simulink subsystem "BLDC_qd_coords"  (R2024a)
settings: Solver=VariableStepAuto  StartTime=0.0  StopTime=10.0  RelTol=1e-3
values from neighbouring files (symbols this model uses):
  Dm = 1e-4    (= 0.0001)    [BLDC_Parameters.m]
  Jt = 1e-3    (= 0.001)    [BLDC_Parameters.m]
  lambda_m = torque_const/(3*P/4)    (= 0.00985)    [BLDC_Parameters.m]
  Lss = Lls + 1.5*Lms    (= 0.0006125)    [BLDC_Parameters.m]
  P = 8    [BLDC_Parameters.m]
  rs = 0.69/2    (= 0.345)    [BLDC_Parameters.m]
  tau_s = 1.06e-3    (= 0.00106)    [BLDC_Parameters.m]
settings Model: Creator=matthewhasman  LastModifiedBy=matthewhasman

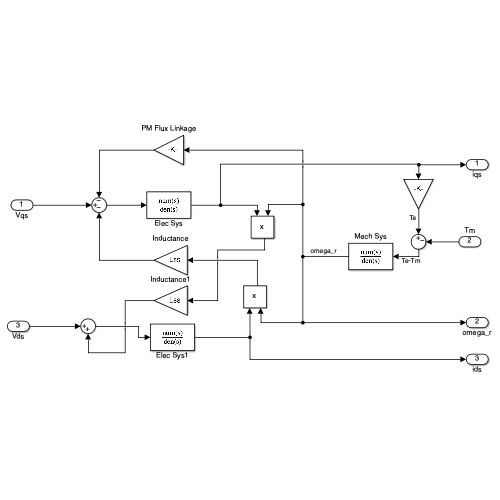
[thumbnail: Simulink's stored preview of the top-level diagram]
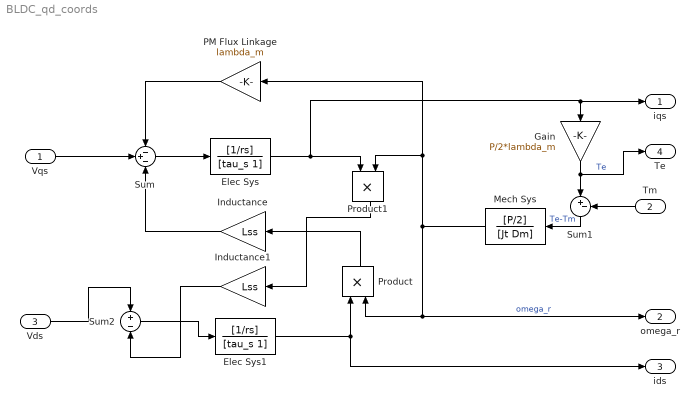
== system BLDC_qd_coords ==
  Vqs : Inport
  Tm : Inport  Port=2
  Vds : Inport  Port=3
  Elec Sys : TransferFcn  Numerator=[1/rs]  Denominator=[tau_s 1]
  Elec Sys1 : TransferFcn  Numerator=[1/rs]  Denominator=[tau_s 1]
  Gain : Gain  Gain=P/2*lambda_m
  Inductance : Gain  Gain=Lss
  Inductance1 : Gain  Gain=Lss
  Mech Sys : TransferFcn  Numerator=[P/2]  Denominator=[Jt Dm]
  PM Flux Linkage : Gain  Gain=lambda_m
  Product : Product
  Product1 : Product
  Sum : Sum  Inputs=-+-
  Sum1 : Sum  Inputs=|+-
  Sum2 : Sum  Inputs=+-
  iqs : Outport
  omega_r : Outport  Port=2
  ids : Outport  Port=3
  Te : Outport  Port=4
  wires:
  Sum/1 -> Elec Sys/1
  Vqs/1 -> Sum/2
  PM Flux Linkage/1 -> Sum/1
  Mech Sys/1 -> Product1/2, PM Flux Linkage/1, omega_r/1, Product/2  "omega_r"
  Inductance/1 -> Sum/3
  Product/1 -> Inductance/1
  Elec Sys/1 -> Product1/1, iqs/1, Gain/1
  Gain/1 -> Sum1/1, Te/1  "Te"
  Tm/1 -> Sum1/2
  Sum1/1 -> Mech Sys/1  "Te-Tm"
  Vds/1 -> Sum2/1
  Product1/1 -> Inductance1/1
  Inductance1/1 -> Sum2/2
  Sum2/1 -> Elec Sys1/1
  Elec Sys1/1 -> Product/1, ids/1
